simulink model "LimitChecking_Gradient"  (R2014a)
settings: Solver=FixedStepDiscrete  StartTime=0.0  StopTime=inf  FixedStep=SampleTime  RelTol=1e-3
InitFcn:
  | limit_gradient = 1;
libraries: simulink x1
settings Model: Creator=georg  LastModifiedBy=georg

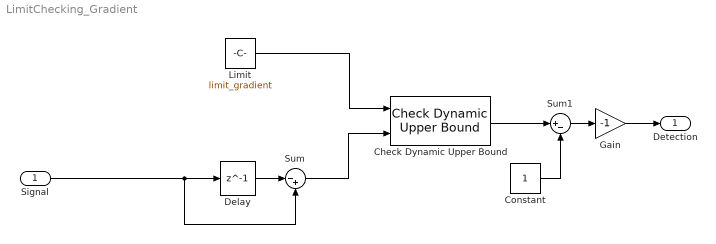
== system LimitChecking_Gradient ==
  Signal : Inport
  Check Dynamic Upper Bound : simulink/Model Verification/Check Dynamic  Upper Bound  Description=sig < max  enabled=on  stopWhenAssertionFail=off  export=on  icon=graphic
  Constant : Constant
  Delay : Delay  DelayLength=1  InitialCondition=0
  Gain : Gain  Gain=-1
  Limit : Constant  Value=limit_gradient
  Sum : Sum  Inputs=|-+
  Sum1 : Sum  Inputs=|+-
  Detection : Outport
  wires:
  Delay/1 -> Sum/1
  Check Dynamic Upper Bound/1 -> Sum1/1
  Sum/1 -> Check Dynamic Upper Bound/2
  Limit/1 -> Check Dynamic Upper Bound/1
  Constant/1 -> Sum1/2
  Sum1/1 -> Gain/1
  Gain/1 -> Detection/1
  Signal/1 -> Sum/2, Delay/1
